simulink model "case_3_model"  (R2025a)
settings: Solver=VariableStepAuto  StartTime=0.0  StopTime=0.1  RelTol=1e-3
libraries: spsPower3phInstantaneousLib x1, spsThreePhaseDynamicLoadLib x1, spsThreePhaseParallelRLCLoadLib x1, spsThreePhaseSeriesRLCBranchLib x1, spsThreePhaseVIMeasurementLib x1, spsThreePhaseSourceLib x1, sps_lib x1
settings Model: Creator=hp  LastModifiedBy=hp
settings DataIOCC: ReturnWorkspaceOutputs=off

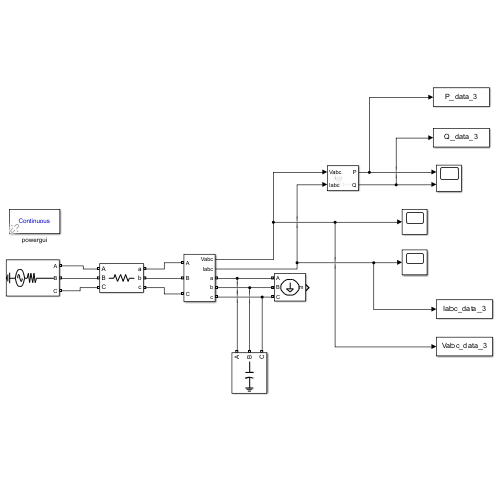
[thumbnail: Simulink's stored preview of the top-level diagram]
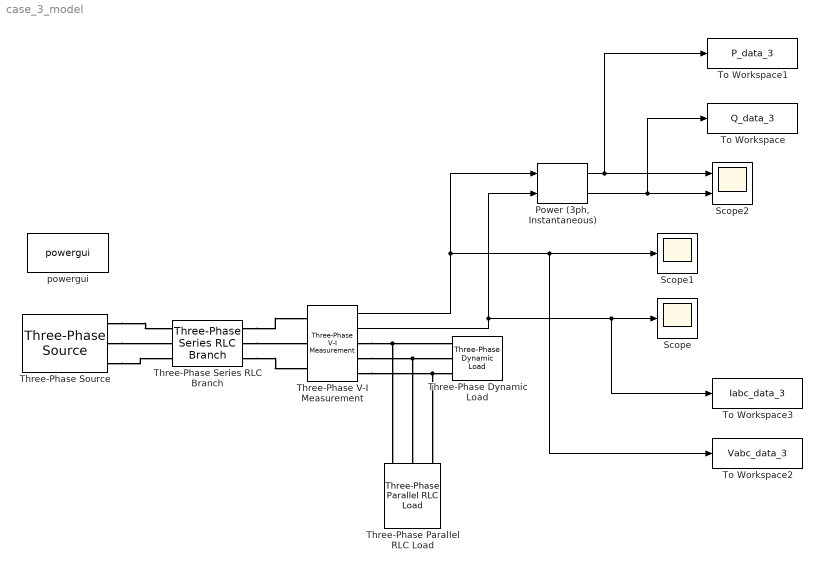
== system case_3_model ==
  "Power (3ph, Instantaneous)" : spsPower3phInstantaneousLib/Power (3ph, Instantaneous)
  Scope : Scope
      settings: ActiveDisplayYMinimum=-86.264898231874213  ActiveDisplayYMaximum=95.922703244769764
  Scope1 : Scope
      settings: ActiveDisplayYMinimum=-386.93627060601864  ActiveDisplayYMaximum=386.91627171119455
  Scope2 : Scope  NumInputPorts=2
      settings: ActiveDisplayYMinimum=4501.838954764542  ActiveDisplayYMaximum=34506.606762398042  DataLoggingVariableName=ScopeData2
  Three-Phase Dynamic Load : spsThreePhaseDynamicLoadLib/Three-Phase Dynamic Load  NominalVoltage=[ 380 50 ]  ActiveReactivePowers=[30000 22500]  PositiveSequence=[1 0]  ExternalControl=off  NpNq=[0 0]  TimeConstants="[0  0  0  0]"  MinimumVoltage=0.7  Tfilter=1e-4  LoadFlowParameters=[4,0,0,0,0]
      settings: LibrarySourceBlock=|
      | sps_lib/Passives/Three-Phase
      | Dynamic Load
  Three-Phase Parallel RLC Load : spsThreePhaseParallelRLCLoadLib/Three-Phase Parallel RLC Load  LConnTagsString=A|B|C  Configuration=Y (grounded)  NominalVoltage=380  Vabc=[1e3 1e3 1e3]  Vabcp=[1e3 1e3 1e3]  NominalFrequency=50  UnbalancedPower=off  ActivePower=0  InductivePower=0  CapacitivePower=12640  Pabc=[10e3 9e3 11e3]  QLabc=[100 90 110]  QCabc=[100 90 110]  Pabcp=[10e3 9e3 11e3]  QLabcp=[100 90 110]  QCabcp=[100 90 110]  Measurements=None  LoadType=constant Z
  Three-Phase Series RLC Branch : spsThreePhaseSeriesRLCBranchLib/Three-Phase Series RLC Branch  LConnTagsString=A|B|C  RConnTagsString=A|B|C  BranchType=R  Resistance=0.01  Inductance=1e-6  Capacitance=1e-6  Measurements=None
  Three-Phase V-I Measurement : spsThreePhaseVIMeasurementLib/Three-Phase V-I Measurement  VoltageMeasurement=phase-to-ground  SetLabelV=off  LabelV=Vabc  Vpu=off  VpuLL=off  CurrentMeasurement=yes  SetLabelI=off  LabelI=Iabc  Ipu=off  Pbase=100e6  Vbase=500e3  OutputType=Complex  PhasorSimulation=off  PSBequivalent=0
  Three-Phase Source : spsThreePhaseSourceLib/Three-Phase Source  InternalConnection=Yg  VoltagePhases=off  Voltage=380  PhaseAngle=0  Voltage_phases=[25e3 25e3 25e3]/sqrt(3)  PhaseAngles_phases=[0 -120 +120]  Frequency=50  NonIdealSource=on  SpecifyImpedance=off  Resistance=0.001  Inductance=0  ShortCircuitLevel=100e6  BaseVoltage=380  XRratio=7  BusType=swing  Pref=10e3  Qref=0  Prefabc=[10e3, 10e3, 10e3]  Qrefabc=[0, 0, 0]  Qmin=-inf  Qmax=inf
  To Workspace : ToWorkspace  VariableName=Q_data_3  SaveFormat=Structure With Time  SampleTime=-1
  To Workspace1 : ToWorkspace  VariableName=P_data_3  SaveFormat=Structure With Time  SampleTime=-1
  To Workspace2 : ToWorkspace  VariableName=Vabc_data_3  SaveFormat=Structure With Time  SampleTime=-1
  To Workspace3 : ToWorkspace  VariableName=Iabc_data_3  SaveFormat=Structure With Time  SampleTime=-1
  powergui : sps_lib/powergui  Priority=1  SimulationMode=Continuous  SampleTime=50e-6  frequency=60  Iterations=50  frequencyindice=50  Pbase=100e6  ErrMax=1e-4  UnitsV=kV  UnitsW=MW  buscounter=0  FunctionMessages=off  echomessages=off  EnableUseOfTLC=off  CurrentSourceSwitches=off  DisableSnubberDevices=off  DisableRonSwitches=off  DisableVfSwitches=off  DisplayEquations=off  AutomaticDiscreteSolvers=off  SolverType=Tustin/Backward Euler (TBE)  Interpol=off  ExternalGateDelay=off  methode=off  Ts=100  x0status=blocks  SPID=on  SwTol=0  HookPort=off  NonlinearTolerance=1e-4  nMaxIteration=100  ContinueOnMaxIteration=off  RestoreLinks=warning  ResistiveCurrentMeasurement=off  Frange=[0:2:500]  Ylog=off  Xlog=on  ShowGrid=off  save=off  variable=ZData  structure=0  ZoomFFT=off  StartTime=0.0  cycles=1  DisplayStyle=1  fundamental=60  FreqAxis=off  MaxFrequency=1000  frequencyindicesteady=1  RmsSteady=1  display=off
  wires:
  Three-Phase V-I Measurement/2 -> "Power (3ph, Instantaneous)"/2, To Workspace3/1, Scope/1
  "Power (3ph, Instantaneous)"/2 -> To Workspace/1, Scope2/2
  Three-Phase V-I Measurement/1 -> "Power (3ph, Instantaneous)"/1, To Workspace2/1, Scope1/1
  "Power (3ph, Instantaneous)"/1 -> To Workspace1/1, Scope2/1
  connections:
  Three-Phase Source/RConn1 -- Three-Phase Series RLC Branch/LConn1
  Three-Phase Source/RConn2 -- Three-Phase Series RLC Branch/LConn2
  Three-Phase Series RLC Branch/RConn2 -- Three-Phase V-I Measurement/LConn2
  Three-Phase V-I Measurement/RConn1 -- Three-Phase Parallel RLC Load/LConn1 -- Three-Phase Dynamic Load/LConn1
  Three-Phase Source/RConn3 -- Three-Phase Series RLC Branch/LConn3
  Three-Phase V-I Measurement/RConn2 -- Three-Phase Parallel RLC Load/LConn2 -- Three-Phase Dynamic Load/LConn2
  Three-Phase V-I Measurement/RConn3 -- Three-Phase Parallel RLC Load/LConn3 -- Three-Phase Dynamic Load/LConn3
  Three-Phase Series RLC Branch/RConn3 -- Three-Phase V-I Measurement/LConn3
  Three-Phase Series RLC Branch/RConn1 -- Three-Phase V-I Measurement/LConn1
